simulink library "BatSense"  (R2017b)
settings: Solver=VariableStepAuto  StartTime=0.0  StopTime=10.0  RelTol=1e-3
settings Model: Creator=sharo  LastModifiedBy=Sharonnie
settings CodeAppCC: StateflowObjectComments=on

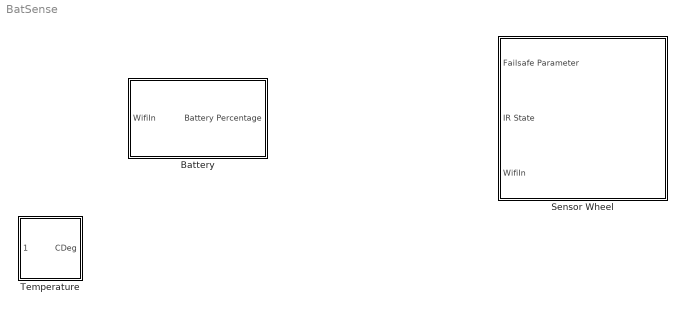
== system BatSense ==
  Battery : Subsystem
  Sensor Wheel : Subsystem
  Temperature : Subsystem

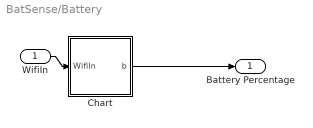
== system BatSense/Battery ==
  WifiIn : Inport
  Chart : Stateflow chart  TreatAsAtomicUnit=on
  Battery Percentage : Outport
  wires:
  WifiIn/1 -> Chart/1(WifiIn)
  Chart/1(b) -> Battery Percentage/1

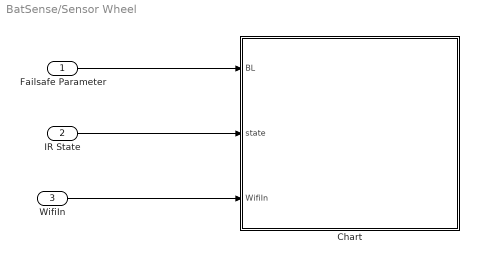
== system BatSense/Sensor Wheel ==
  Failsafe Parameter : Inport
  IR State : Inport  Port=2
  WifiIn : Inport  Port=3
  Chart : Stateflow chart  TreatAsAtomicUnit=on
  wires:
  IR State/1 -> Chart/2(state)
  Failsafe Parameter/1 -> Chart/1(BL)
  WifiIn/1 -> Chart/3(WifiIn)

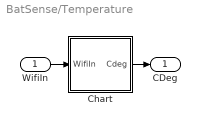
== system BatSense/Temperature ==
  WifiIn : Inport
  Chart : Stateflow chart  TreatAsAtomicUnit=on
  CDeg : Outport
  wires:
  WifiIn/1 -> Chart/1(WifiIn)
  Chart/1(Cdeg) -> CDeg/1

== stateflow chart BatSense/Battery/Chart ==
  state Bat
    en,du:
    battery= BatterySense;
    b = battery'
  (default) -> Bat
  data: h function_output; WifiIn input; b output; battery local
  function h = BatterySense:
    | function h = BatterySense
    | h = [0,0,0];
    | persistent obi
    | 
    | coder.extrinsic('evalin');
    | coder.extrinsic('BatteryChargeReaderRoomba');
    | coder.extrinsic('get');
    | 
    | 
    | if isempty(obi);
    |     obi=evalin('base','so');
    | end
    | 
    | h = BatteryChargeReaderRoomba(obi)

== stateflow chart BatSense/Temperature/Chart ==
  state Celcius
    entry,during:
    Cdeg = T;
  (default) -> Celcius
  data: t function_output; Cdeg output; WifiIn input
  function t = T:
    | function t = T
    | persistent obi
    | t =1;
    | coder.extrinsic('evalin');
    | coder.extrinsic('TemperatureRoomba');
    | coder.extrinsic('get');
    | 
    | temp=0;
    | 
    |     obi = evalin('base','so');
    | 
    | temp=TemperatureRoomba(obi);
    | 
    | t=temp;

== stateflow chart BatSense/Sensor Wheel/Chart ==
  state LogicBox
    state Failsafe
      entry: WheelCtrl(0,0);
    state Power
      state Reverse
        entry:
        WheelCtrl(.3,.3)
      state Forward
        entry:
        WheelCtrl(.25, .25);
      state Sensor4
        entry:
        WheelCtrl(.35, .2)
      state Sensor6
        entry:
        WheelCtrl(.25, .1)
      state Sensor2
        entry:
        WheelCtrl(-.15, .3)
      state Sensor3
        entry:
        WheelCtrl(-.2, .35)
      state Sensor5
        entry:
        WheelCtrl(.3, -.15)
      state Sensor1
        entry:
        WheelCtrl (-.1, .25)
      (default) -> Reverse
      Reverse -> Forward : [after(2,sec)]
      Forward -> Sensor1 [order 1] : [state(1)==1]
      Sensor1 -> Forward : [state(1)<1]
      Forward -> Sensor2 [order 2] : [state(2)==1]
      Sensor2 -> Forward : [state(2)<1]
      Forward -> Sensor3 [order 3] : [state(3)==1]
      Sensor3 -> Forward : [state(3)<1]
      Forward -> Sensor4 [order 4] : [state(4)==1]
      Sensor4 -> Forward : [state(4)<1]
      Forward -> Sensor5 [order 5] : [state(5)==1]
      Sensor5 -> Forward : [state(5)<1]
      Forward -> Sensor6 [order 6] : [state(6)==1]
      Sensor6 -> Forward : [state(6)<1]
    (default) -> Failsafe
    Failsafe -> Power : [BL<15]
    Power -> Failsafe : [BL>=15]
  (default) -> LogicBox
  data: rw function_input; lw function_input; BL input; state input; WifiIn input
  function WheelCtrl(rw,lw):
    | function WheelCtrl(rw,lw)
    | persistent obi
    | coder.extrinsic('evalin');
    | coder.extrinsic('get');
    | coder.extrinsic('SetWheelVelRoomba');
    | 
    | if isempty(obi);
    | obi = evalin('base','so');
    | 
    | end
    | 
    | SetWheelVelRoomba(obi,rw,lw);
